simulink model "LABA_CONTINOUS"  (R2023a)
settings: Solver=VariableStepAuto  StartTime=0.0  StopTime=10  RelTol=1e-3
model workspace: external: MAT-File C:\Users\Jasminis\OneDrive\S7003E\LABA_CONT.mat (data not in the file)
values from neighbouring files (symbols this model uses):
  A = [0 0 0 0 1 -435.034344762 0 1903.43949265 0 -6.0990753006 0 62.0192858703 ... (16 elements, 4x4)]    [LABA_CONT.mat]    (also in LABA_CONT_PARAMETERS.m = zeros(4); LabA3_3.m = zeros(4))
  B = [0  0; 20.5759487388  -5.37234378316; 0  0; -90.0275435714  31.1948458246]    [LABA_CONT.mat]    (also in LABA_CONT_PARAMETERS.m = zeros(4,2); LabA3_3.m = zeros(4,1))
  C = [1 0 0 0 0 1 0 0 0 0 1 0 ... (16 elements, 4x4)]    [LABA_CONT.mat]    (also in LABA_CONT_PARAMETERS.m = eye(4); LabA3_3.m = [ 0 0 1 0])
  D = [0  0; 0  0; 0  0; 0  0]    [LABA_CONT.mat]    (also in LABA_CONT_PARAMETERS.m = zeros(4,2); LabA3_3.m = 0)
  Kd = -1.57156122147    [LABA_CONT.mat]
  Ki = -52940.0364782    [LABA_CONT.mat]
  Kp = -858.036557676    [LABA_CONT.mat]
  Ts = 0.00122562104376    [LABA_CONT.mat]
libraries: slpidlib x1, SignalEditorBlockLib x1
settings Model: Creator=Jasminis  LastModifiedBy=Jasminis

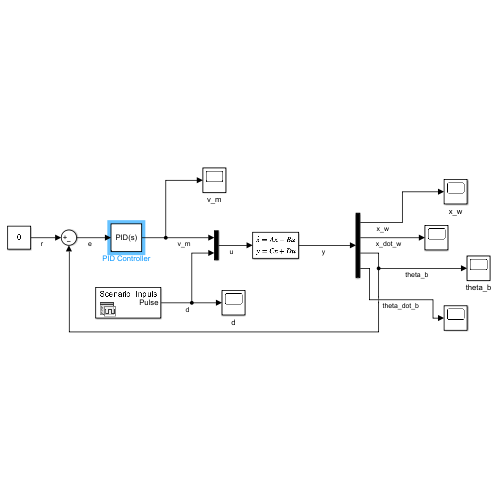
[thumbnail: Simulink's stored preview of the top-level diagram]
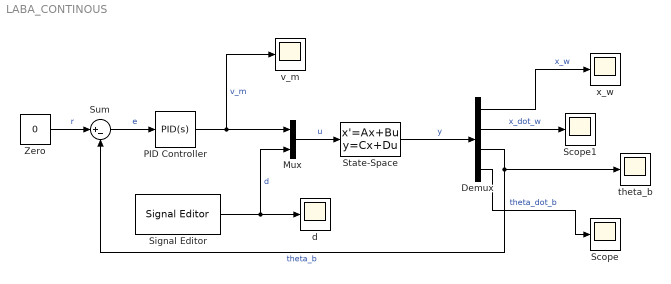
== system LABA_CONTINOUS ==
  Demux : Demux
  Mux : Mux  Inputs=2
  PID Controller : slpidlib/PID Controller  Controller=PID  Form=Parallel  TimeDomain=Continuous-time  UseExternalTs=off  SampleTime=Ts  IntegratorMethod=Forward Euler  FilterMethod=Forward Euler  ControllerParametersSource=internal  P=Kp  I=Ki  UseKiTs=off  D=Kd  N=1000  UseFilter=on  TunerSelectOption=Transfer Function Based (PID Tuner App)  InitialConditionSource=internal  InitialConditionForIntegrator=0  InitialConditionForFilter=0  DifferentiatorICPrevScaledInput=0  ExternalReset=none  TrackingMode=off  Kt=1  LimitOutput=off  SatLimitsSource=internal  UpperSaturationLimit=inf  LowerSaturationLimit=-inf  LinearizeAsGain=on  AntiWindupMode=none  Kb=1  LimitIntegrator=off  UpperIntegratorSaturationLimit=inf  LowerIntegratorSaturationLimit=-inf  POutMin=[]  POutMax=[]  IOutMin=[]  IOutMax=[]  DOutMin=[]  DOutMax=[]  NOutMin=[]  NOutMax=[]  SumOutMin=[]  SumOutMax=[]  SaturationOutMin=[]  SaturationOutMax=[]  PParamMin=[]  PParamMax=[]  IParamMin=[]  IParamMax=[]  DParamMin=[]  DParamMax=[]  NParamMin=[]  NParamMax=[]  KbParamMin=[]  KbParamMax=[]  KtParamMin=[]  KtParamMax=[]  KbOutMin=[]  KbOutMax=[]  KtOutMin=[]  KtOutMax=[]  IntegratorOutMin=[]  IntegratorOutMax=[]  FilterOutMin=[]  FilterOutMax=[]  SumI1OutMin=[]  SumI1OutMax=[]  SumI2OutMin=[]  SumI2OutMax=[]  SumI3OutMin=[]  SumI3OutMax=[]  SumI4OutMin=[]  SumI4OutMax=[]  SumDOutMin=[]  SumDOutMax=[]  DifferentiatorOutMin=[]  DifferentiatorOutMax=[]  FilterDiffOutCoefMin=[]  FilterDiffOutCoefMax=[]  ReciprocalOutMin=[]  ReciprocalOutMax=[]  SumDenOutMin=[]  SumDenOutMax=[]  SumNumOutMin=[]  SumNumOutMax=[]  DivideOutMin=[]  DivideOutMax=[]  UdiffTsProdOutMin=[]  UdiffTsProdOutMax=[]  NTsProdOutMin=[]  NTsProdOutMax=[]  UintegralTsProdOutMin=[]  UintegralTsProdOutMax=[]  UngainTsProdOutMin=[]  UngainTsProdOutMax=[]  ClampingZeroOutDataTypeStr=Inherit: Inherit via back propagation  ClampingZeroOutMin=[]  ClampingZeroOutMax=[]  FilterDenConstantOutDataTypeStr=Inherit: Inherit via back propagation  FilterDenConstantOutMin=[]  FilterDenConstantOutMax=[]  PCopyOutDataTypeStr=Inherit: Inherit via back propagation  PCopyOutMin=[]  PCopyOutMax=[]  NCopyOutDataTypeStr=Inherit: Inherit via back propagation  NCopyOutMin=[]  NCopyOutMax=[]  IntegratorContinuousStateAttributes=''  IntegratorStateMustResolveToSignalObject=off  IntegratorRTWStateStorageClass=Auto  FilterContinuousStateAttributes=''  FilterStateMustResolveToSignalObject=off  FilterRTWStateStorageClass=Auto  ParallelPVariant=InternalParameters  IdealPVariant=Disabled  IVariant=InternalParameters  DVariant=InternalParameters  IntegratorVariant=Continuous  SatVariant=Disabled  AWVariant=Passthrough  PCopyVariant=Disabled  TRVariant=Disabled  FdbkBlocksVariant=Forward  IdealPFdbkVariant=Disabled  SatFdbkVariant=Disabled  DerivativeFilterVariant=ContFilter  NVariant=InternalParameters  NCopyVariant=Disabled  FilterICVariant=InternalICsFilter  IntegratorICVariant=InternalICs  ExternalResetVariant=Disabled  TRSumVariant=Passthrough  SumFdbkVariant=Disabled  SumVariant=Sum_PID  TsampFilterVariant=InternalTs  TsampNgainVariant=Passthrough  TsampIntegralVariant=Disabled_SignalSpec  ExternalSaturationOutDataTypeStr=Inherit: Same as second input
  Scope : Scope
  Scope1 : Scope
  Signal Editor : SignalEditorBlockLib/Signal Editor  FileName=pulse.mat  ActiveScenario=Scenario_Inpuls  ActiveSignal=Pulse  IsBus=off  OutputBusObjectStr=Bus: BusObject  SampleTime=0  Interpolate=off  ZeroCross=off  OutputAfterFinalValue=Setting to zero  Unit=inherit  PreserveSignalName=on  ApplySigPropsToAllScenarios=on
  State-Space : StateSpace  A=A  B=B  C=C  D=D  InitialCondition=0  ParameterTunability=Unconstrained
  Sum : Sum  Inputs=|+-
  Zero : Constant  Value=0  OutDataTypeStr=Inherit: Inherit via back propagation
  d : Scope
  theta_b : Scope
  v_m : Scope
  x_w : Scope
  wires:
  State-Space/1 -> Demux/1  "y"
  Mux/1 -> State-Space/1  "u"
  Demux/1 -> x_w/1  "x_w"
  Demux/3 -> Sum/2, theta_b/1  "theta_b"
  PID Controller/1 -> v_m/1, Mux/1  "v_m"
  Signal Editor/1 -> Mux/2, d/1  "d"
  Zero/1 -> Sum/1  "r"
  Sum/1 -> PID Controller/1  "e"
  Demux/4 -> Scope/1  "theta_dot_b"
  Demux/2 -> Scope1/1  "x_dot_w"
